simulink model "VMC_LateralTrajectoryPlanningControllerV04"  (R2018b)
settings: Solver=FixedStepDiscrete  StartTime=0.0  StopTime=10  FixedStep=0.02  RelTol=1e-3
values from neighbouring files (symbols this model uses):
  D_d_end = 0    [TRP_parameters.m]
  P_optimizer_interations = 5.0    (= 5)    [TRP_parameters.m]
  P_TRP_Lat_dT = 0.02    [TRP_parameters.m]
  P_Vehicle_width = 1.8    [TRP_parameters.m]
  P_vVeh_min_TrajCalc = 5.0    (= 5)    [TRP_parameters.m]
libraries: simulink x1
(part 1 of 2)
settings Model: Creator=qiand  LastModifiedBy=qiand

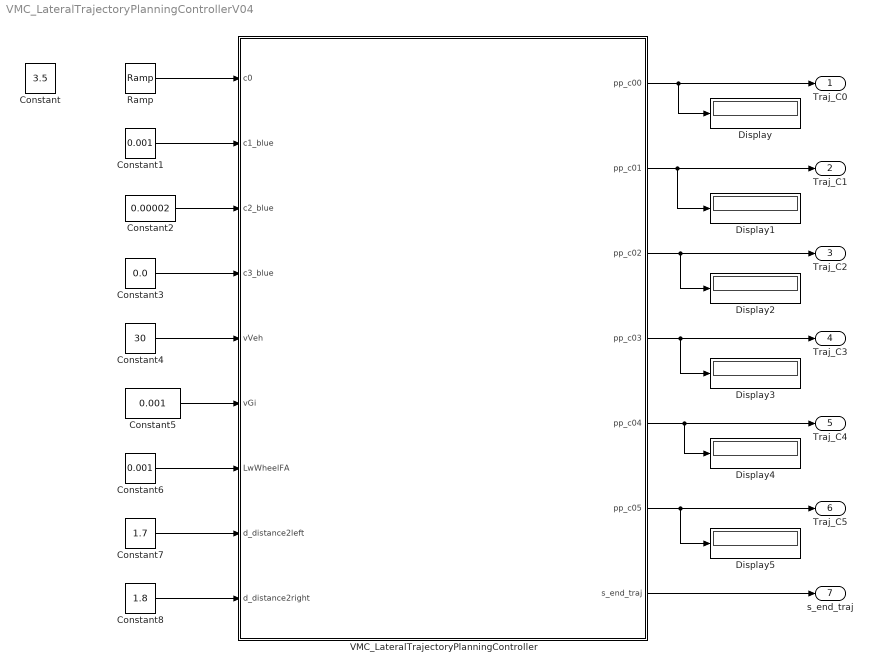
== system VMC_LateralTrajectoryPlanningControllerV04 ==
  Constant : Constant  Value=3.5
  Constant1 : Constant  Value=0.001
  Constant2 : Constant  Value=0.00002
  Constant3 : Constant  Value=0.0
  Constant4 : Constant  Value=30
  Constant5 : Constant  Value=0.001
  Constant6 : Constant  Value=0.001
  Constant7 : Constant  Value=1.7
  Constant8 : Constant  Value=1.8
  Display{,1..5} (6 alike) : Display
  Ramp : simulink/Sources/Ramp  slope=-0.35  start=0  InitialOutput=3.5
  VMC_LateralTrajectoryPlanningController : Subsystem
  Traj_C0 : Outport
  Traj_C1 : Outport  Port=2
  Traj_C2 : Outport  Port=3
  Traj_C3 : Outport  Port=4
  Traj_C4 : Outport  Port=5
  Traj_C5 : Outport  Port=6
  s_end_traj : Outport  Port=7
  wires:
  VMC_LateralTrajectoryPlanningController/1(pp_c00) -> Display/1, Traj_C0/1
  VMC_LateralTrajectoryPlanningController/2(pp_c01) -> Display1/1, Traj_C1/1
  VMC_LateralTrajectoryPlanningController/3(pp_c02) -> Display2/1, Traj_C2/1
  VMC_LateralTrajectoryPlanningController/4(pp_c03) -> Display3/1, Traj_C3/1
  VMC_LateralTrajectoryPlanningController/5(pp_c04) -> Display4/1, Traj_C4/1
  VMC_LateralTrajectoryPlanningController/6(pp_c05) -> Display5/1, Traj_C5/1
  VMC_LateralTrajectoryPlanningController/7(s_end_traj) -> s_end_traj/1
  Constant1/1 -> VMC_LateralTrajectoryPlanningController/2(c1_blue)
  Constant2/1 -> VMC_LateralTrajectoryPlanningController/3(c2_blue)
  Constant3/1 -> VMC_LateralTrajectoryPlanningController/4(c3_blue)
  Constant4/1 -> VMC_LateralTrajectoryPlanningController/5(vVeh)
  Constant5/1 -> VMC_LateralTrajectoryPlanningController/6(vGi)
  Constant6/1 -> VMC_LateralTrajectoryPlanningController/7(LwWheelFA)
  Constant7/1 -> VMC_LateralTrajectoryPlanningController/8(d_distance2left)
  Constant8/1 -> VMC_LateralTrajectoryPlanningController/9(d_distance2right)
  Ramp/1 -> VMC_LateralTrajectoryPlanningController/1(c0)

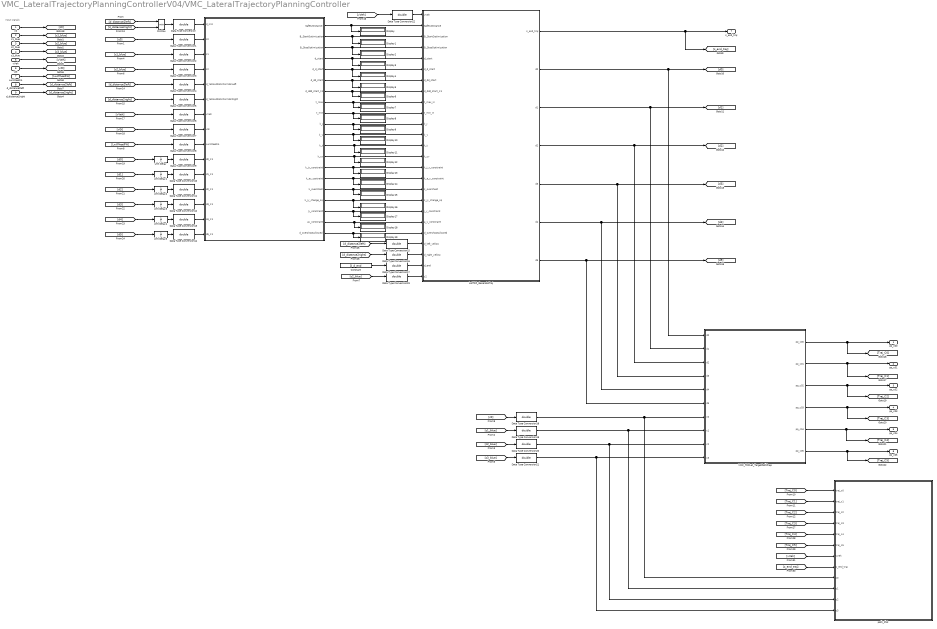
== system VMC_LateralTrajectoryPlanningControllerV04/VMC_LateralTrajectoryPlanningController ==
  note: Input signals
  c0 : Inport
  c1_blue : Inport  Port=2
  c2_blue : Inport  Port=3
  c3_blue : Inport  Port=4
  vVeh : Inport  Port=5
  vGi : Inport  Port=6
  LwWheelFA : Inport  Port=7
  d_distance2left : Inport  Port=8
  d_distance2right : Inport  Port=9
  "  " : Subsystem
  Constant : Constant  Value=D_d_end
  Data Type Conversion{,1..23} (24 alike) : DataTypeConversion  OutDataTypeStr=double
  Display{,1..19} (20 alike) : Display
  LatTRP_GenerateTraj : Subsystem
  MinMax : MinMax  Inputs=2
  Unit Delay{,1..5} (6 alike) : UnitDelay  SampleTime=-1
  VMC_TRPLat_TargetPathPrep : Subsystem
  path_Plot : Subsystem
  pp_c00 : Outport
  pp_c01 : Outport  Port=2
  pp_c02 : Outport  Port=3
  pp_c03 : Outport  Port=4
  pp_c04 : Outport  Port=5
  pp_c05 : Outport  Port=6
  s_end_traj : Outport  Port=7
  wires:
  d_distance2left/1 -> [d_distance2left]
  c0/1 -> [c0]
  LwWheelFA/1 -> [LwWheelFA]
  c2_blue/1 -> [c2_blue]
  vGi/1 -> [vGi]
  d_distance2right/1 -> [d_distance2right]
  c3_blue/1 -> [c3_blue]
  c1_blue/1 -> [c1_blue]
  vVeh/1 -> [vVeh]
  MinMax/1 -> Data Type Conversion/1
  [d_distance2right] -> Data Type Conversion5/1
  Unit Delay1/1 -> Data Type Conversion10/1
  [d0] -> Unit Delay/1
  Unit Delay3/1 -> Data Type Conversion12/1
  [d_distance2left] -> MinMax/1
  [c2_blue] -> Data Type Conversion3/1
  [c1_blue] -> Data Type Conversion2/1
  Unit Delay4/1 -> Data Type Conversion13/1
  [d4] -> Unit Delay4/1
  [vGi] -> Data Type Conversion7/1
  [d_distance2right] -> MinMax/2
  Unit Delay/1 -> Data Type Conversion9/1
  [d3] -> Unit Delay3/1
  [d1] -> Unit Delay1/1
  [d2] -> Unit Delay2/1
  Unit Delay2/1 -> Data Type Conversion11/1
  [vVeh] -> Data Type Conversion6/1
  [LwWheelFA] -> Data Type Conversion8/1
  [c0] -> Data Type Conversion1/1
  [d5] -> Unit Delay5/1
  Unit Delay5/1 -> Data Type Conversion14/1
  [d_distance2left] -> Data Type Conversion4/1
  Data Type Conversion/1 -> "  "/1(d_min)
  Data Type Conversion1/1 -> "  "/2(c0)
  Data Type Conversion2/1 -> "  "/3(c1)
  Data Type Conversion3/1 -> "  "/4(c2)
  Data Type Conversion4/1 -> "  "/5(d_YellowStaticCorridorLeft)
  Data Type Conversion5/1 -> "  "/6(d_YellowStaticCorridorRight)
  Data Type Conversion6/1 -> "  "/7(vVeh)
  Data Type Conversion7/1 -> "  "/8(vGi)
  Data Type Conversion8/1 -> "  "/9(LwWheelFA)
  Data Type Conversion9/1 -> "  "/10(d0_K1)
  Data Type Conversion10/1 -> "  "/11(d1_K1)
  Data Type Conversion11/1 -> "  "/12(d2_K1)
  Data Type Conversion12/1 -> "  "/13(d3_K1)
  Data Type Conversion13/1 -> "  "/14(d4_K1)
  Data Type Conversion14/1 -> "  "/15(d5_K1)
  LatTRP_GenerateTraj/6(d4) -> VMC_TRPLat_TargetPathPrep/5(d4), [d4]
  VMC_TRPLat_TargetPathPrep/3(pp_c02) -> pp_c02/1, [Traj_C2]
  [c2_blue] -> Data Type Conversion20/1
  VMC_TRPLat_TargetPathPrep/1(pp_c00) -> [Traj_C0], pp_c00/1
  [d_distance2left] -> Data Type Conversion15/1
  [c1_blue] -> Data Type Conversion19/1
  VMC_TRPLat_TargetPathPrep/5(pp_c04) -> [Traj_C4], pp_c04/1
  LatTRP_GenerateTraj/2(d0) -> VMC_TRPLat_TargetPathPrep/1(d0), [d0]
  Constant/1 -> Data Type Conversion17/1
  VMC_TRPLat_TargetPathPrep/4(pp_c03) -> [Traj_C3], pp_c03/1
  [vVeh] -> Data Type Conversion22/1
  [c3_blue] -> Data Type Conversion21/1
  [d_distance2right] -> Data Type Conversion16/1
  LatTRP_GenerateTraj/1(s_end_traj) -> [s_end_traj], s_end_traj/1
  VMC_TRPLat_TargetPathPrep/2(pp_c01) -> [Traj_C1], pp_c01/1
  [c0] -> Data Type Conversion18/1
  LatTRP_GenerateTraj/5(d3) -> VMC_TRPLat_TargetPathPrep/4(d3), [d3]
  LatTRP_GenerateTraj/7(d5) -> VMC_TRPLat_TargetPathPrep/6(d5), [d5]
  LatTRP_GenerateTraj/4(d2) -> VMC_TRPLat_TargetPathPrep/3(d2), [d2]
  LatTRP_GenerateTraj/3(d1) -> VMC_TRPLat_TargetPathPrep/2(d1), [d1]
  VMC_TRPLat_TargetPathPrep/6(pp_c05) -> [Traj_C5], pp_c05/1
  "  "/1(SafetyDistance) -> Display/1, LatTRP_GenerateTraj/2(SafetyDistance)
  "  "/2(B_StartOptimization) -> Display1/1, LatTRP_GenerateTraj/3(B_StartOptimization)
  "  "/3(B_StopOptimization) -> Display2/1, LatTRP_GenerateTraj/4(B_StopOptimization)
  "  "/4(d_start) -> Display3/1, LatTRP_GenerateTraj/5(d_start)
  "  "/5(d_d_start) -> Display4/1, LatTRP_GenerateTraj/6(d_d_start)
  "  "/6(d_dd_start) -> Display5/1, LatTRP_GenerateTraj/7(d_dd_start)
  "  "/7(d_ddd_start_k1) -> Display6/1, LatTRP_GenerateTraj/8(d_ddd_start_K1)
  "  "/8(t_max) -> Display7/1, LatTRP_GenerateTraj/9(t_max_in)
  "  "/9(t_min) -> Display8/1, LatTRP_GenerateTraj/10(t_min_in)
  "  "/10(k_j) -> Display9/1, LatTRP_GenerateTraj/11(k_j)
  "  "/11(k_v) -> Display10/1, LatTRP_GenerateTraj/12(k_v)
  "  "/12(k_t) -> Display11/1, LatTRP_GenerateTraj/13(k_t)
  "  "/13(k_cv) -> Display12/1, LatTRP_GenerateTraj/14(k_cv)
  "  "/14(k_jy_constraint) -> Display13/1, LatTRP_GenerateTraj/15(k_j_y_constraint)
  "  "/15(k_ay_costraint) -> Display14/1, LatTRP_GenerateTraj/16(k_a_y_constraint)
  "  "/16(k_overshoot) -> Display15/1, LatTRP_GenerateTraj/17(k_overshoot)
  "  "/17(k_jy_change_sq) -> Display16/1, LatTRP_GenerateTraj/18(k_jy_change_sq)
  "  "/18(jy_constraint) -> Display17/1, LatTRP_GenerateTraj/19(j_y_constraint)
  "  "/19(ay_constraint) -> Display18/1, LatTRP_GenerateTraj/20(a_y_constraint)
  "  "/20(d_overshootAllowed) -> Display19/1, LatTRP_GenerateTraj/21(d_overshootAllowed)
  Data Type Conversion15/1 -> LatTRP_GenerateTraj/22(d_left_yellow)
  Data Type Conversion16/1 -> LatTRP_GenerateTraj/23(d_right_yellow)
  Data Type Conversion17/1 -> LatTRP_GenerateTraj/24(d_end)
  Data Type Conversion18/1 -> path_Plot/9(c0), VMC_TRPLat_TargetPathPrep/7(c0)
  Data Type Conversion19/1 -> path_Plot/10(c1), VMC_TRPLat_TargetPathPrep/8(c1)
  Data Type Conversion20/1 -> path_Plot/11(c2), VMC_TRPLat_TargetPathPrep/9(c2)
  Data Type Conversion21/1 -> path_Plot/12(c3), VMC_TRPLat_TargetPathPrep/10(c3)
  Data Type Conversion22/1 -> LatTRP_GenerateTraj/1(vVeh)
  [c2_blue] -> Data Type Conversion23/1
  Data Type Conversion23/1 -> LatTRP_GenerateTraj/25(c2)
  [vVeh] -> path_Plot/7(vVeh)
  [s_end_traj] -> path_Plot/8(s_end_traj)
  [Traj_C0] -> path_Plot/1(traj_c0)
  [Traj_C1] -> path_Plot/2(traj_c1)
  [Traj_C2] -> path_Plot/3(traj_c2)
  [Traj_C3] -> path_Plot/4("traj_c3 ")
  [Traj_C4] -> path_Plot/5(traj_c4)
  [Traj_C5] -> path_Plot/6(traj_c5)

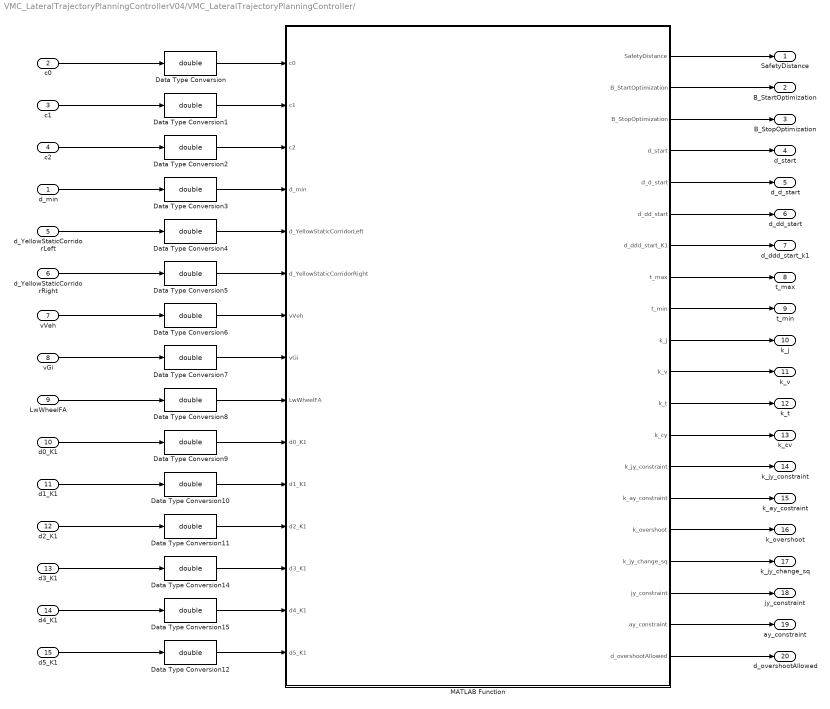
== system VMC_LateralTrajectoryPlanningControllerV04/VMC_LateralTrajectoryPlanningController/   ==
  d_min : Inport
  c0 : Inport  Port=2
  c1 : Inport  Port=3
  c2 : Inport  Port=4
  d_YellowStaticCorridorLeft : Inport  Port=5
  d_YellowStaticCorridorRight : Inport  Port=6
  vVeh : Inport  Port=7
  vGi : Inport  Port=8
  LwWheelFA : Inport  Port=9
  d0_K1 : Inport  Port=10
  d1_K1 : Inport  Port=11
  d2_K1 : Inport  Port=12
  d3_K1 : Inport  Port=13
  d4_K1 : Inport  Port=14
  d5_K1 : Inport  Port=15
  Data Type Conversion{,1..12,14..15} (15 alike) : DataTypeConversion  OutDataTypeStr=double
  MATLAB Function : MATLAB Function  TreatAsAtomicUnit=on
  SafetyDistance : Outport
  B_StartOptimization : Outport  Port=2
  B_StopOptimization : Outport  Port=3
  d_start : Outport  Port=4
  d_d_start : Outport  Port=5
  d_dd_start : Outport  Port=6
  d_ddd_start_k1 : Outport  Port=7
  t_max : Outport  Port=8
  t_min : Outport  Port=9
  k_j : Outport  Port=10
  k_v : Outport  Port=11
  k_t : Outport  Port=12
  k_cv : Outport  Port=13
  k_jy_constraint : Outport  Port=14
  k_ay_costraint : Outport  Port=15
  k_overshoot : Outport  Port=16
  k_jy_change_sq : Outport  Port=17
  jy_constraint : Outport  Port=18
  ay_constraint : Outport  Port=19
  d_overshootAllowed : Outport  Port=20
  wires:
  MATLAB Function/20(d_overshootAllowed) -> d_overshootAllowed/1
  MATLAB Function/19(ay_constraint) -> ay_constraint/1
  MATLAB Function/18(jy_constraint) -> jy_constraint/1
  MATLAB Function/17(k_jy_change_sq) -> k_jy_change_sq/1
  MATLAB Function/16(k_overshoot) -> k_overshoot/1
  MATLAB Function/15(k_ay_constraint) -> k_ay_costraint/1
  MATLAB Function/14(k_jy_constraint) -> k_jy_constraint/1
  MATLAB Function/13(k_cy) -> k_cv/1
  MATLAB Function/1(SafetyDistance) -> SafetyDistance/1
  MATLAB Function/2(B_StartOptimization) -> B_StartOptimization/1
  MATLAB Function/3(B_StopOptimization) -> B_StopOptimization/1
  MATLAB Function/4(d_start) -> d_start/1
  MATLAB Function/5(d_d_start) -> d_d_start/1
  MATLAB Function/6(d_dd_start) -> d_dd_start/1
  MATLAB Function/7(d_ddd_start_K1) -> d_ddd_start_k1/1
  MATLAB Function/8(t_max) -> t_max/1
  MATLAB Function/9(t_min) -> t_min/1
  MATLAB Function/10(k_j) -> k_j/1
  MATLAB Function/11(k_v) -> k_v/1
  MATLAB Function/12(k_t) -> k_t/1
  c0/1 -> Data Type Conversion/1
  c1/1 -> Data Type Conversion1/1
  c2/1 -> Data Type Conversion2/1
  d_min/1 -> Data Type Conversion3/1
  d_YellowStaticCorridorLeft/1 -> Data Type Conversion4/1
  d_YellowStaticCorridorRight/1 -> Data Type Conversion5/1
  vVeh/1 -> Data Type Conversion6/1
  vGi/1 -> Data Type Conversion7/1
  LwWheelFA/1 -> Data Type Conversion8/1
  d0_K1/1 -> Data Type Conversion9/1
  d1_K1/1 -> Data Type Conversion10/1
  d2_K1/1 -> Data Type Conversion11/1
  d3_K1/1 -> Data Type Conversion14/1
  d4_K1/1 -> Data Type Conversion15/1
  d5_K1/1 -> Data Type Conversion12/1
  Data Type Conversion/1 -> MATLAB Function/1(c0)
  Data Type Conversion1/1 -> MATLAB Function/2(c1)
  Data Type Conversion2/1 -> MATLAB Function/3(c2)
  Data Type Conversion3/1 -> MATLAB Function/4(d_min)
  Data Type Conversion4/1 -> MATLAB Function/5(d_YellowStaticCorridorLeft)
  Data Type Conversion5/1 -> MATLAB Function/6(d_YellowStaticCorridorRight)
  Data Type Conversion6/1 -> MATLAB Function/7(vVeh)
  Data Type Conversion7/1 -> MATLAB Function/8(vGi)
  Data Type Conversion8/1 -> MATLAB Function/9(LwWheelFA)
  Data Type Conversion9/1 -> MATLAB Function/10(d0_K1)
  Data Type Conversion10/1 -> MATLAB Function/11(d1_K1)
  Data Type Conversion11/1 -> MATLAB Function/12(d2_K1)
  Data Type Conversion15/1 -> MATLAB Function/14(d4_K1)
  Data Type Conversion12/1 -> MATLAB Function/15(d5_K1)
  Data Type Conversion14/1 -> MATLAB Function/13(d3_K1)

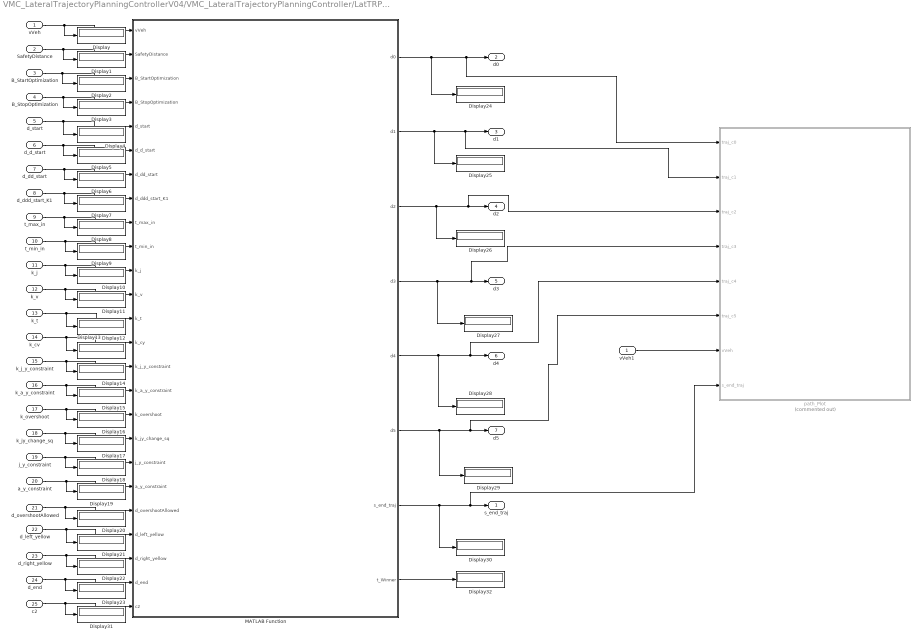
== system VMC_LateralTrajectoryPlanningControllerV04/VMC_LateralTrajectoryPlanningController/LatTRP_GenerateTraj ==
  vVeh : Inport
  SafetyDistance : Inport  Port=2
  B_StartOptimization : Inport  Port=3
  B_StopOptimization : Inport  Port=4
  d_start : Inport  Port=5
  d_d_start : Inport  Port=6
  d_dd_start : Inport  Port=7
  d_ddd_start_K1 : Inport  Port=8
  t_max_in : Inport  Port=9
  t_min_in : Inport  Port=10
  k_j : Inport  Port=11
  k_v : Inport  Port=12
  k_t : Inport  Port=13
  k_cv : Inport  Port=14
  k_j_y_constraint : Inport  Port=15
  k_a_y_constraint : Inport  Port=16
  k_overshoot : Inport  Port=17
  k_jy_change_sq : Inport  Port=18
  j_y_constraint : Inport  Port=19
  a_y_constraint : Inport  Port=20
  d_overshootAllowed : Inport  Port=21
  d_left_yellow : Inport  Port=22
  d_right_yellow : Inport  Port=23
  d_end : Inport  Port=24
  c2 : Inport  Port=25
  Display{,1..32} (33 alike) : Display
  MATLAB Function : MATLAB Function  TreatAsAtomicUnit=on
  path_Plot : Subsystem  Commented=on
  vVeh1 : InportShadow
  s_end_traj : Outport
  d0 : Outport  Port=2
  d1 : Outport  Port=3
  d2 : Outport  Port=4
  d3 : Outport  Port=5
  d4 : Outport  Port=6
  d5 : Outport  Port=7
  wires:
  d_right_yellow/1 -> Display22/1, MATLAB Function/23(d_right_yellow)
  d_end/1 -> MATLAB Function/24(d_end), Display23/1
  d_left_yellow/1 -> Display21/1, MATLAB Function/22(d_left_yellow)
  a_y_constraint/1 -> Display19/1, MATLAB Function/20(a_y_constraint)
  j_y_constraint/1 -> Display18/1, MATLAB Function/19(j_y_constraint)
  k_jy_change_sq/1 -> Display17/1, MATLAB Function/18(k_jy_change_sq)
  d_start/1 -> Display4/1, MATLAB Function/5(d_start)
  vVeh/1 -> Display/1, MATLAB Function/1(vVeh)
  B_StopOptimization/1 -> Display3/1, MATLAB Function/4(B_StopOptimization)
  SafetyDistance/1 -> Display1/1, MATLAB Function/2(SafetyDistance)
  B_StartOptimization/1 -> Display2/1, MATLAB Function/3(B_StartOptimization)
  k_overshoot/1 -> Display16/1, MATLAB Function/17(k_overshoot)
  d_dd_start/1 -> Display6/1, MATLAB Function/7(d_dd_start)
  d_d_start/1 -> Display5/1, MATLAB Function/6(d_d_start)
  d_ddd_start_K1/1 -> Display7/1, MATLAB Function/8(d_ddd_start_K1)
  k_a_y_constraint/1 -> Display15/1, MATLAB Function/16(k_a_y_constraint)
  k_v/1 -> Display11/1, MATLAB Function/12(k_v)
  k_j/1 -> Display10/1, MATLAB Function/11(k_j)
  k_j_y_constraint/1 -> Display14/1, MATLAB Function/15(k_j_y_constraint)
  k_t/1 -> Display12/1, MATLAB Function/13(k_t)
  k_cv/1 -> Display13/1, MATLAB Function/14(k_cy)
  t_max_in/1 -> Display8/1, MATLAB Function/9(t_max_in)
  t_min_in/1 -> Display9/1, MATLAB Function/10(t_min_in)
  MATLAB Function/1(d0) -> path_Plot/1(traj_c0), d0/1, Display24/1
  MATLAB Function/2(d1) -> path_Plot/2(traj_c1), d1/1, Display25/1
  MATLAB Function/3(d2) -> Display26/1, path_Plot/3(traj_c2), d2/1
  MATLAB Function/4(d3) -> Display27/1, path_Plot/4("traj_c3 "), d3/1
  MATLAB Function/5(d4) -> Display28/1, path_Plot/5(traj_c4), d4/1
  MATLAB Function/6(d5) -> Display29/1, path_Plot/6(traj_c5), d5/1
  MATLAB Function/7(s_end_traj) -> Display30/1, path_Plot/8(s_end_traj), s_end_traj/1
  c2/1 -> MATLAB Function/25(c2), Display31/1
  MATLAB Function/8(t_Winner) -> Display32/1
  d_overshootAllowed/1 -> Display20/1, MATLAB Function/21(d_overshootAllowed)
  vVeh1/1 -> path_Plot/7(vVeh)

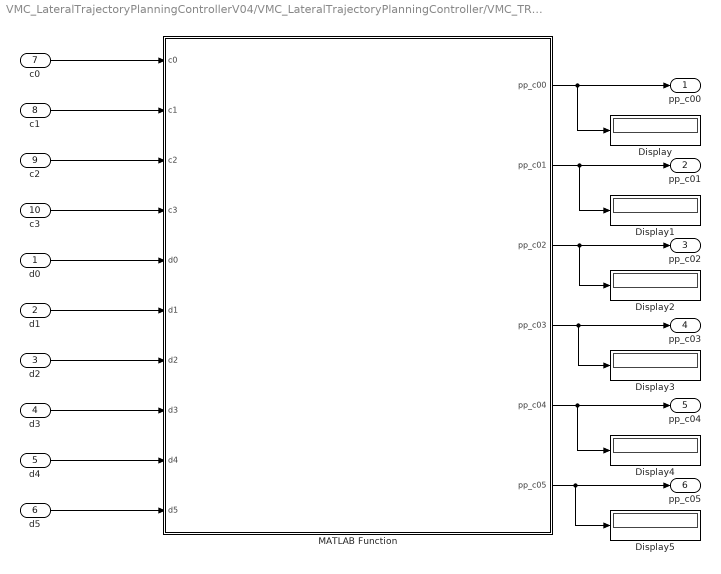
== system VMC_LateralTrajectoryPlanningControllerV04/VMC_LateralTrajectoryPlanningController/VMC_TRPLat_TargetPathPrep ==
  d0 : Inport
  d1 : Inport  Port=2
  d2 : Inport  Port=3
  d3 : Inport  Port=4
  d4 : Inport  Port=5
  d5 : Inport  Port=6
  c0 : Inport  Port=7
  c1 : Inport  Port=8
  c2 : Inport  Port=9
  c3 : Inport  Port=10
  Display{,1..5} (6 alike) : Display
  MATLAB Function : MATLAB Function  TreatAsAtomicUnit=on
  pp_c00 : Outport
  pp_c01 : Outport  Port=2
  pp_c02 : Outport  Port=3
  pp_c03 : Outport  Port=4
  pp_c04 : Outport  Port=5
  pp_c05 : Outport  Port=6
  wires:
  c0/1 -> MATLAB Function/1(c0)
  c1/1 -> MATLAB Function/2(c1)
  c2/1 -> MATLAB Function/3(c2)
  c3/1 -> MATLAB Function/4(c3)
  d0/1 -> MATLAB Function/5(d0)
  d1/1 -> MATLAB Function/6(d1)
  d2/1 -> MATLAB Function/7(d2)
  d3/1 -> MATLAB Function/8(d3)
  MATLAB Function/1(pp_c00) -> Display/1, pp_c00/1
  MATLAB Function/5(pp_c04) -> Display4/1, pp_c04/1
  MATLAB Function/3(pp_c02) -> Display2/1, pp_c02/1
  MATLAB Function/2(pp_c01) -> Display1/1, pp_c01/1
  MATLAB Function/4(pp_c03) -> Display3/1, pp_c03/1
  MATLAB Function/6(pp_c05) -> Display5/1, pp_c05/1
  d4/1 -> MATLAB Function/9(d4)
  d5/1 -> MATLAB Function/10(d5)

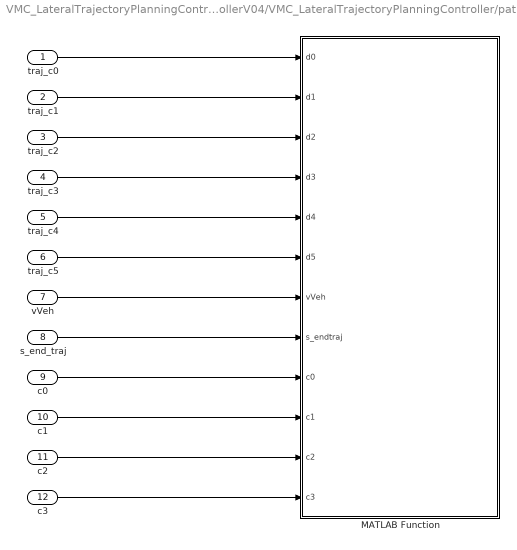
== system VMC_LateralTrajectoryPlanningControllerV04/VMC_LateralTrajectoryPlanningController/path_Plot ==
  traj_c0 : Inport
  traj_c1 : Inport  Port=2
  traj_c2 : Inport  Port=3
  "traj_c3 " : Inport  Port=4
  traj_c4 : Inport  Port=5
  traj_c5 : Inport  Port=6
  vVeh : Inport  Port=7
  s_end_traj : Inport  Port=8
  c0 : Inport  Port=9
  c1 : Inport  Port=10
  c2 : Inport  Port=11
  c3 : Inport  Port=12
  MATLAB Function : MATLAB Function  TreatAsAtomicUnit=on
  wires:
  traj_c0/1 -> MATLAB Function/1(d0)
  traj_c2/1 -> MATLAB Function/3(d2)
  traj_c1/1 -> MATLAB Function/2(d1)
  "traj_c3 "/1 -> MATLAB Function/4(d3)
  traj_c4/1 -> MATLAB Function/5(d4)
  traj_c5/1 -> MATLAB Function/6(d5)
  vVeh/1 -> MATLAB Function/7(vVeh)
  s_end_traj/1 -> MATLAB Function/8(s_endtraj)
  c0/1 -> MATLAB Function/9(c0)
  c1/1 -> MATLAB Function/10(c1)
  c2/1 -> MATLAB Function/11(c2)
  c3/1 -> MATLAB Function/12(c3)

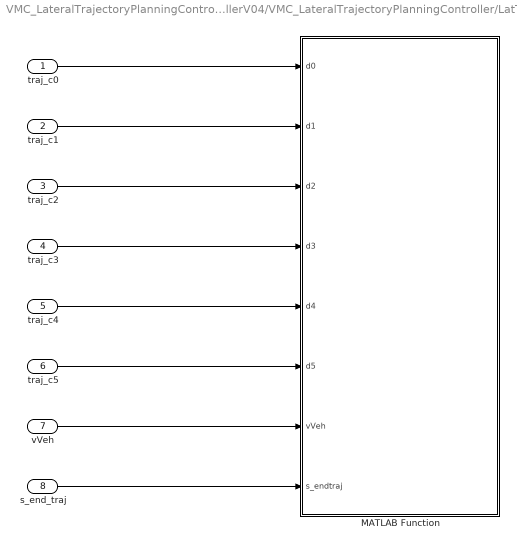
== system VMC_LateralTrajectoryPlanningControllerV04/VMC_LateralTrajectoryPlanningController/LatTRP_GenerateTraj/path_Plot ==
  traj_c0 : Inport
  traj_c1 : Inport  Port=2
  traj_c2 : Inport  Port=3
  "traj_c3 " : Inport  Port=4
  traj_c4 : Inport  Port=5
  traj_c5 : Inport  Port=6
  vVeh : Inport  Port=7
  s_end_traj : Inport  Port=8
  MATLAB Function : MATLAB Function  TreatAsAtomicUnit=on
  wires:
  traj_c0/1 -> MATLAB Function/1(d0)
  traj_c2/1 -> MATLAB Function/3(d2)
  traj_c1/1 -> MATLAB Function/2(d1)
  "traj_c3 "/1 -> MATLAB Function/4(d3)
  traj_c4/1 -> MATLAB Function/5(d4)
  traj_c5/1 -> MATLAB Function/6(d5)
  vVeh/1 -> MATLAB Function/7(vVeh)
  s_end_traj/1 -> MATLAB Function/8(s_endtraj)

== matlab function VMC_LateralTrajectoryPlanningControllerV04/VMC_LateralTrajectoryPlanningController/LatTRP_GenerateTraj/path_Plot/MATLAB Function ==
  data: d0 input; d1 input; d2 input; d3 input; d4 input; d5 input; vVeh input; s_endtraj input
function fcn(d0, d1, d2, d3, d4, d5, vVeh, s_endtraj)

dist_x = d0 : s_endtraj;
dist_y = d0 + d1 * dist_x + d2 * dist_x.^2 + d3 * dist_x.^3 + d4 * dist_x.^4 + d5 * dist_x.^5 ;
handles = plot(dist_x, dist_y, 'r');
pause (0.01);
grid on 
% hold on

== matlab function VMC_LateralTrajectoryPlanningControllerV04/VMC_LateralTrajectoryPlanningController/path_Plot/MATLAB Function ==
  data: d0 input; d1 input; d2 input; d3 input; d4 input; d5 input; vVeh input; s_endtraj input; c0 input; c1 input; c2 input; c3 input
function fcn(d0, d1, d2, d3, d4, d5, vVeh, s_endtraj, c0,c1, c2, c3)

x= 0 : s_endtraj;
y = d0 + d1 * x + d2 * x.^2 + d3 * x.^3 + d4 * x.^4 + d5 * x.^5;
y1 = c0 + c1 * x + c2 * x.^2 + c3 * x.^3;
handles = plot(x,y1,'b');
% hold on
handles = plot(x,y,'r');
hold on 
 pause (0.01);
%axis([0,s_endtraj ,-0.5,4])

== matlab function VMC_LateralTrajectoryPlanningControllerV04/VMC_LateralTrajectoryPlanningController/  /MATLAB Function ==
  data: SafetyDistance output; c0 input; c1 input; c2 input; d_min input; d_YellowStaticCorridorLeft input; d_YellowStaticCorridorRight input; vVeh input; vGi input; LwWheelFA input; d0_K1 input; d1_K1 input; d2_K1 input; d3_K1 input; d4_K1 input; d5_K1 input; B_StartOptimization output; B_StopOptimization output; d_start output; d_d_start output; d_dd_start output; d_ddd_start_K1 output; t_max output; t_min output; k_j output; k_v output; k_t output; k_cy output; k_jy_constraint output; k_ay_constraint output; k_overshoot output; k_jy_change_sq output; jy_constraint output; ay_constraint output; d_overshootAllowed output; P_TRP_Lat_ay_constraint_comfort parameter; P_TRP_lat_d_overshootAllowed_comfort parameter; P_TRP_Lat_dT parameter; P_TRP_Lat_jy_constraint_comfort parameter; P_TRP_Lat_k_ay_constraint_comfort parameter; P_TRP_Lat_k_j_comfort parameter; P_TRP_Lat_k_jy_change_sq_comfort parameter; P_TRP_Lat_k_jy_constraint_comfort parameter; P_TRP_Lat_k_overshoot_comfort parameter; P_TRP_Lat_k_t_comfort parameter; P_TRP_Lat_k_t_mod_d_comfort_CurX parameter; P_TRP_Lat_k_t_mod_d_comfort_CurY parameter; P_TRP_Lat_tPredDistToPosConstraint parameter; P_TRP_Lat_k_v_comfort parameter; P_TRP_Lat_vVehiMinYawRate parameter; P_TRP_Lat_k_v_mod_d_comfort_CurX parameter; P_TRP_Lat_k_v_mod_d_comfort_CurY parameter; P_TRP_Lat_k_v_mod_d_min_comfort_CurX parameter; P_TRP_Lat_k_v_mod_d_min_comfort_CurY parameter; P_TRP_Lat_SafetyDistance_comfort parameter; P_TRP_Lat_SafetyDistance_emergency parameter; P_TRP_Lat_startUpTime parameter; P_TRP_Lat_vVeh_min_TrajCalc parameter; P_TRP_Lat_t_max_comfort_CurX parameter; P_TRP_Lat_t_max_comfort_CurY parameter; P_TRP_Lat_t_min_comfort_CurX parameter; P_TRP_Lat_t_min_comfort_CurY parameter; P_TRP_Lat_vy_diff_max_emergency_CurX parameter; P_TRP_Lat_vy_diff_max_emergency_CurY parameter; P_TRP_Lat_ay_diff_max_emergency_CurX parameter; P_TRP_Lat_ay_diff_max_emergency_CurY parameter; lx_WheelBase parameter; P_Vehicle_width parameter; P_TRP_Lat_y_diff_max_emergency_CurX parameter; P_TRP_Lat_y_diff_max_emergency_CurY parameter; P_TRP_Lat_k_cy_Comfort parameter; P_TRP_Lat_k_j_mod_d_comfort_CurX parameter; P_TRP_Lat_k_j_mod_d_comfort_CurY parameter; P_TRP_Lat_k_t_mod_d_min_comfort_CurX parameter; P_TRP_Lat_k_t_mod_d_min_comfort_CurY parameter; P_TRP_Lat_k_j_mod_d_min_comfort_CurX parameter; P_TRP_Lat_k_j_mod_d_min_comfort_CurY parameter
function [SafetyDistance,B_StartOptimization,B_StopOptimization,...
          d_start,d_d_start,d_dd_start,d_ddd_start_K1,t_max,t_min,k_j,k_v,k_t,k_cy,...
          k_jy_constraint,k_ay_constraint,k_overshoot,k_jy_change_sq,... 
          jy_constraint,ay_constraint,d_overshootAllowed]= fcn(c0,c1,c2,d_min,d_YellowStaticCorridorLeft,d_YellowStaticCorridorRight,...
                                                               vVeh,vGi,LwWheelFA,d0_K1,d1_K1,d2_K1,d3_K1,d4_K1,d5_K1,...
                                                               P_TRP_Lat_ay_constraint_comfort,P_TRP_lat_d_overshootAllowed_comfort,P_TRP_Lat_dT,...
                                                               P_TRP_Lat_jy_constraint_comfort,P_TRP_Lat_k_ay_constraint_comfort,...
                                                               P_TRP_Lat_k_j_comfort,P_TRP_Lat_k_jy_change_sq_comfort,...
                                                               P_TRP_Lat_k_jy_constraint_comfort,P_TRP_Lat_k_overshoot_comfort,...
                                                               P_TRP_Lat_k_t_comfort,P_TRP_Lat_k_t_mod_d_comfort_CurX,P_TRP_Lat_k_t_mod_d_comfort_CurY,P_TRP_Lat_tPredDistToPosConstraint,...
                                                               P_TRP_Lat_k_v_comfort,P_TRP_Lat_vVehiMinYawRate,...
                                                               P_TRP_Lat_k_v_mod_d_comfort_CurX,P_TRP_Lat_k_v_mod_d_comfort_CurY,...
                                                               P_TRP_Lat_k_v_mod_d_min_comfort_CurX,P_TRP_Lat_k_v_mod_d_min_comfort_CurY,...
                                                               P_TRP_Lat_SafetyDistance_comfort,P_TRP_Lat_SafetyDistance_emergency,P_TRP_Lat_startUpTime,P_TRP_Lat_vVeh_min_TrajCalc,...
                                                               P_TRP_Lat_t_max_comfort_CurX,P_TRP_Lat_t_max_comfort_CurY,...
                                                               P_TRP_Lat_t_min_comfort_CurX,P_TRP_Lat_t_min_comfort_CurY,...
                                                               P_TRP_Lat_vy_diff_max_emergency_CurX,P_TRP_Lat_vy_diff_max_emergency_CurY,P_TRP_Lat_ay_diff_max_emergency_CurX,P_TRP_Lat_ay_diff_max_emergency_CurY,...
                                                               lx_WheelBase,P_Vehicle_width,P_TRP_Lat_y_diff_max_emergency_CurX,P_TRP_Lat_y_diff_max_emergency_CurY,P_TRP_Lat_k_cy_Comfort,...
                                                               P_TRP_Lat_k_j_mod_d_comfort_CurX,P_TRP_Lat_k_j_mod_d_comfort_CurY,P_TRP_Lat_k_t_mod_d_min_comfort_CurX,P_TRP_Lat_k_t_mod_d_min_comfort_CurY,...
                                                               P_TRP_Lat_k_j_mod_d_min_comfort_CurX,P_TRP_Lat_k_j_mod_d_min_comfort_CurY)

D_ay_constraint_comfort = P_TRP_Lat_ay_constraint_comfort;

D_ay_diff_max_emergency_CurX = P_TRP_Lat_ay_diff_max_emergency_CurX;
D_ay_diff_max_emergency_CurY = P_TRP_Lat_ay_diff_max_emergency_CurY;
D_d_overshootAllowed_comfort = P_TRP_lat_d_overshootAllowed_comfort;
D_dT = P_TRP_Lat_dT;
D_jy_constraint_comfort = P_TRP_Lat_jy_constraint_comfort;
D_k_ay_constraint_comfort = P_TRP_Lat_k_ay_constraint_comfort;
D_k_cy_Comfort = P_TRP_Lat_k_cy_Comfort;
D_k_j_comfort = P_TRP_Lat_k_j_comfort;
D_k_j_mod_d_comfort_CurX = P_TRP_Lat_k_j_mod_d_comfort_CurX;
D_k_j_mod_d_comfort_CurY = P_TRP_Lat_k_j_mod_d_comfort_CurY;
D_k_j_mod_d_min_comfort_CurX = P_TRP_Lat_k_j_mod_d_min_comfort_CurX;
D_k_j_mod_d_min_comfort_CurY = P_TRP_Lat_k_j_mod_d_min_comfort_CurY;
D_k_jy_change_sq_comfort = P_TRP_Lat_k_jy_change_sq_comfort;
D_k_jy_constraint_comfort = P_TRP_Lat_k_jy_constraint_comfort;
D_k_overshoot_comfort = P_TRP_Lat_k_overshoot_comfort;
D_k_t_comfort = P_TRP_Lat_k_t_comfort;
D_k_t_mod_d_comfort_CurX = P_TRP_Lat_k_t_mod_d_comfort_CurX;
D_k_t_mod_d_comfort_CurY = P_TRP_Lat_k_t_mod_d_comfort_CurY;
D_k_t_mod_d_min_comfort_CurX = P_TRP_Lat_k_t_mod_d_min_comfort_CurX;
D_k_t_mod_d_min_comfort_CurY = P_TRP_Lat_k_t_mod_d_min_comfort_CurY;
D_k_v_comfort = P_TRP_Lat_k_v_comfort;
D_k_v_mod_d_comfort_CurX = P_TRP_Lat_k_v_mod_d_comfort_CurX;
D_k_v_mod_d_comfort_CurY = P_TRP_Lat_k_v_mod_d_comfort_CurY;
D_k_v_mod_d_min_comfort_CurX = P_TRP_Lat_k_v_mod_d_min_comfort_CurX;
D_k_v_mod_d_min_comfort_CurY = P_TRP_Lat_k_v_mod_d_min_comfort_CurY;
D_SafetyDistance_comfort = P_TRP_Lat_SafetyDistance_comfort;
D_SafetyDistance_emergency = P_TRP_Lat_SafetyDistance_emergency;
D_startUpTime = P_TRP_Lat_startUpTime;
D_t_max_comfort_CurX = P_TRP_Lat_t_max_comfort_CurX;
D_t_max_comfort_CurY = P_TRP_Lat_t_max_comfort_CurY;
D_t_min_comfort_CurX = P_TRP_Lat_t_min_comfort_CurX;
D_t_min_comfort_CurY = P_TRP_Lat_t_min_comfort_CurY;
D_tPredDistToPosConstraint = P_TRP_Lat_tPredDistToPosConstraint;
D_vVeh_min = P_TRP_Lat_vVeh_min_TrajCalc;
D_vVeh_switch2steerAg = P_TRP_Lat_vVehiMinYawRate;
% D_vy_diff_max_comfort = P_TRP_Lat_vy_diff_max_comfort;
D_vy_diff_max_emergency_CurX = P_TRP_Lat_vy_diff_max_emergency_CurX;
D_vy_diff_max_emergency_CurY = P_TRP_Lat_vy_diff_max_emergency_CurY;
D_wheelbase = lx_WheelBase;
% D_y_diff_max_comfort = P_TRP_Lat_y_diff_max_comfort;
D_y_diff_max_emergency_CurX = P_TRP_Lat_y_diff_max_emergency_CurX;
D_y_diff_max_emergency_CurY = P_TRP_Lat_y_diff_max_emergency_CurY;

persistent timeSinceActivation
%persistent delta_s
%persistent delta_s_p2
if isempty(timeSinceActivation)
%    delta_s = 0;
%    delta_s_p2 = 0;
    timeSinceActivation = 0;
end

% limit vehicle longitudinal velocity to not become smaller than D_vVeh_min
vVeh_lim = max( vVeh, D_vVeh_min );  % 5m/s
vVeh_lim_p2 = vVeh_lim * vVeh_lim;

% 0 offset for violation checking with yellow static corridor
% because the trajectory will always be planned for the current timestamp
%s_offset = 0;



if vVeh < D_vVeh_switch2steerAg  % 1m/s
    
    kappa_vehicle_act = LwWheelFA / D_wheelbase;
else
    
    kappa_vehicle_act = vGi / vVeh;
end

% always plan in one cycle for now
B_StartOptimization = true;
B_StopOptimization = true;

% setting start conditions

    delta_s = vVeh * D_dT;
    delta_s_p2 = delta_s * delta_s;
    delta_s_p3 = delta_s_p2 * delta_s;
    delta_s_p4 = delta_s_p3 * delta_s;
    delta_s_p5 = delta_s_p4 * delta_s;
    
    % setting the start boundary conditions for the target path
    d_start = d0_K1 + d1_K1 * delta_s + d2_K1 * delta_s_p2 + d3_K1 * delta_s_p3 + d4_K1 * delta_s_p4 + d5_K1 *delta_s_p5;
    d_d_start = d1_K1 + 2 *d2_K1 * delta_s + 3 * d3_K1 * delta_s_p2 + 4 * d4_K1 * delta_s_p3 + 5 * d5_K1 * delta_s_p4;
    d_dd_start = 2 * d2_K1 + 6 * d3_K1 * delta_s + 12 * d4_K1 * delta_s_p2 + 20 * d5_K1 * delta_s_p3;
    
    % setting the cuvature change of the last target path 
    % used to prevent jumps in the planned curvature change at the start of the target path
    d_ddd_start_K1 = 6 * d3_K1 + 24 * d4_K1 * delta_s + 60 * d5_K1 * delta_s_p2;

% limitation of difference between planned and actual state:
% use parameters for allowed differences
% scale allowed difference on predicted distance to position constraint
% no difference allowed for a certain timespan after activation

    if c0 > 0
        distToPosConstraint = -(c0 + c1 * vVeh * D_tPredDistToPosConstraint) - (d_YellowStaticCorridorRight + 0.5 * P_Vehicle_width + D_SafetyDistance_emergency);
    else
        distToPosConstraint = (c0 + c1 * vVeh * D_tPredDistToPosConstraint) + (d_YellowStaticCorridorLeft - 0.5 * P_Vehicle_width - D_SafetyDistance_emergency);
    end
    y_diff_max = lookforchart(D_y_diff_max_emergency_CurX,D_y_diff_max_emergency_CurY,distToPosConstraint);
    vy_diff_max = lookforchart(D_vy_diff_max_emergency_CurX,D_vy_diff_max_emergency_CurY,distToPosConstraint);
    ay_diff_max = lookforchart(D_ay_diff_max_emergency_CurX,D_ay_diff_max_emergency_CurY,distToPosConstraint);


% calculate timer since activation

    timeSinceActivation = timeSinceActivation + D_dT;

timeSinceActivation = min(timeSinceActivation,100);

% set scaling of state limitation to 0 for a specific time after activation
% after that use the scaling according to the distance to the position
% constraint
if timeSinceActivation < D_startUpTime
    y_diff_max = 0;
    vy_diff_max = 0;
    ay_diff_max = 0;
else
    % keep state limitation as they are set above 
end

% limit start boundary conditions to a value not too far from the current
% vehicle state 
d_start = min(d_start,-c0 + y_diff_max);
d_start = max(d_start,-c0 - y_diff_max);
d_d_start = min(d_d_start,-c1 + vy_diff_max / vVeh_lim);
d_d_start = max(d_d_start,-c1 - vy_diff_max / vVeh_lim);
d_dd_start = min(d_dd_start,kappa_vehicle_act - c2 + ay_diff_max/vVeh_lim_p2);
d_dd_start = max(d_dd_start,kappa_vehicle_act - c2 - ay_diff_max/vVeh_lim_p2);

ay_startCondition = (c2 + d_dd_start) * vVeh_lim_p2;

% set cost weights and dynamic constraints according to behaviour strategy


    k_cy = D_k_cy_Comfort;
    t_min = lookforchart(D_t_min_comfort_CurX,D_t_min_comfort_CurY,abs(d_start));
    t_max = lookforchart(D_t_max_comfort_CurX,D_t_max_comfort_CurY,abs(d_start));
    k_j_mod_d =lookforchart(D_k_j_mod_d_comfort_CurX,D_k_j_mod_d_comfort_CurY,abs(d_start));
    k_v_mod_d =lookforchart(D_k_v_mod_d_comfort_CurX,D_k_v_mod_d_comfort_CurY,abs(d_start));
    k_t_mod_d =lookforchart(D_k_t_mod_d_comfort_CurX,D_k_t_mod_d_comfort_CurY,abs(d_start));
    k_j_mod_d_min =lookforchart(D_k_j_mod_d_min_comfort_CurX,D_k_j_mod_d_min_comfort_CurY,d_min);
    k_v_mod_d_min =lookforchart(D_k_v_mod_d_min_comfort_CurX,D_k_v_mod_d_min_comfort_CurY,d_min);
    k_t_mod_d_min =lookforchart(D_k_t_mod_d_min_comfort_CurX,D_k_t_mod_d_min_comfort_CurY,d_min);
    k_j = k_j_mod_d * k_j_mod_d_min * D_k_j_comfort;
    k_v = k_v_mod_d * k_v_mod_d_min * D_k_v_comfort;
    k_t = k_t_mod_d * k_t_mod_d_min * D_k_t_comfort;
    k_jy_constraint = D_k_jy_constraint_comfort;
    k_ay_constraint = D_k_ay_constraint_comfort;
    k_overshoot = D_k_overshoot_comfort;
    k_jy_change_sq = D_k_jy_change_sq_comfort;
    
    jy_constraint = D_jy_constraint_comfort;
    ay_constraint = max(abs(ay_startCondition),D_ay_constraint_comfort);
    d_overshootAllowed = D_d_overshootAllowed_comfort;
    
    SafetyDistance = D_SafetyDistance_comfort;
